simulink model "one"  (R2020b)
settings: Solver=FixedStepDiscrete  StartTime=0.0  StopTime=200  FixedStep=0.1  RelTol=1e-3  EnableMultiTasking=on
settings Model: Creator=USER  LastModifiedBy=USER

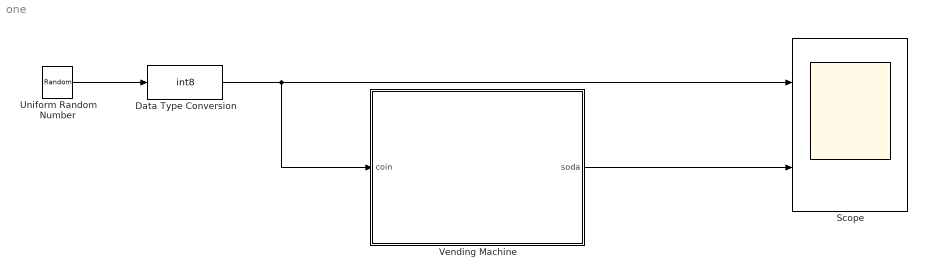
== system one ==
  Data Type Conversion : DataTypeConversion  OutDataTypeStr=int8  RndMeth=Nearest  SaturateOnIntegerOverflow=on
  Scope : Scope  NumInputPorts=2
  Uniform Random Number : UniformRandomNumber  Minimum=0  Maximum=2  Seed=337  SampleTime=10
  Vending Machine : Stateflow chart  TreatAsAtomicUnit=on
  wires:
  Vending Machine/1(soda) -> Scope/2
  Uniform Random Number/1 -> Data Type Conversion/1
  Data Type Conversion/1 -> Scope/1, Vending Machine/1(coin)

== stateflow chart one/Vending Machine ==
  settings: stateMachineType=MEALY_MACHINE  initializeOutput=1
  state Vending
  state Lime
  state Cola
  (default) -> Vending
  Lime -> Vending [order 2] : [coin ==2]{soda=1}
  Vending -> Lime [order 1] : [coin == 1]{soda=0}
  Cola -> Vending [order 1] : [coin==1]{soda=1}
  Vending -> Cola [order 2] : [coin==2]{soda=0}
  Lime -> Cola [order 1] : [coin==1]{soda=0}
  Cola -> Lime [order 2] : [coin==2]{soda=1}
  data: coin input; soda output
